simulink model "plant_1"  (R2017b)
settings: Solver=FixedStepAuto  StartTime=0.0  StopTime=10.0  FixedStep=10e-4
settings Model: Creator=Mehmet  LastModifiedBy=Mehmet

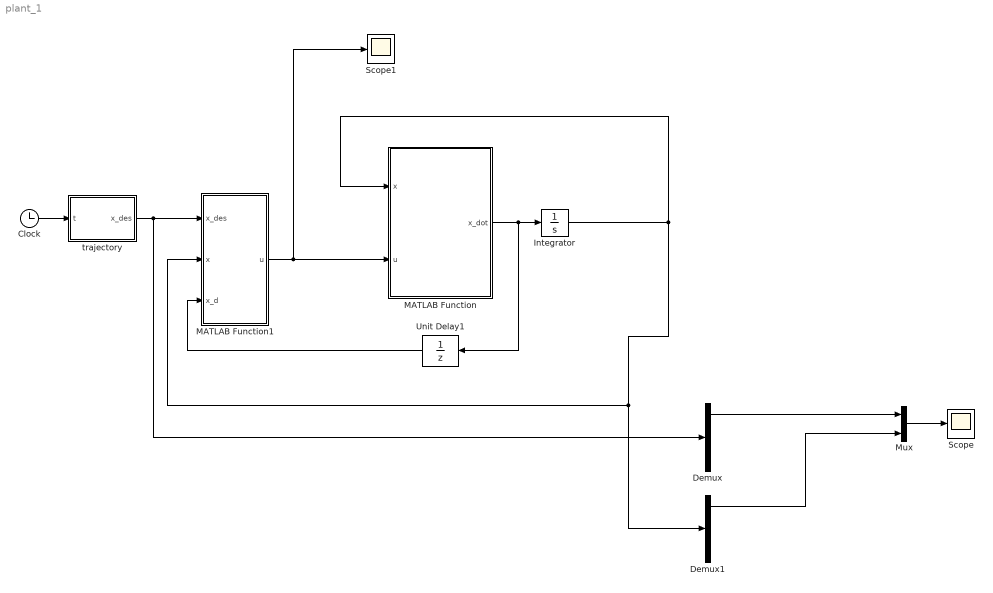
== system plant_1 ==
  Clock : Clock
  Demux : Demux  Outputs=3
  Demux1 : Demux  Outputs=3
  Integrator : Integrator  InitialCondition=[0;0;0]
  MATLAB Function : MATLAB Function  TreatAsAtomicUnit=on
  MATLAB Function1 : MATLAB Function  TreatAsAtomicUnit=on
  Mux : Mux  Inputs=2
  Scope : Scope
  Scope1 : Scope
  Unit Delay1 : UnitDelay  SampleTime=-1
  trajectory : MATLAB Function  TreatAsAtomicUnit=on
  wires:
  MATLAB Function1/1(u) -> Scope1/1, MATLAB Function/2(u)
  Clock/1 -> trajectory/1(t)
  trajectory/1(x_des) -> Demux/1, MATLAB Function1/1(x_des)
  Demux/1 -> Mux/1
  Demux1/1 -> Mux/2
  Mux/1 -> Scope/1
  MATLAB Function/1(x_dot) -> Unit Delay1/1, Integrator/1
  Integrator/1 -> Demux1/1, MATLAB Function1/2(x), MATLAB Function/1(x)
  Unit Delay1/1 -> MATLAB Function1/3(x_d)

== matlab function plant_1/MATLAB Function1 ==
  data: x_des input; u output; x input; x_d input
function u = fcn(x_des,x,x_d)

f_x = sin(x(1)) + x(2)*x(3) + x(1)*x(2)^2;
g_x = 1 + x(1)^2;

Kp = 100;
Kd = 14.14;

% v = y_dd + Kd*e_d + Kp*e;

e = x_des(1) - x(1);
e_d = x_des(2) - x_d(1);

v = x_des(3) + Kd*e_d + Kp*e;

u = 1/g_x*(-f_x + v);

end

== matlab function plant_1/MATLAB Function ==
  data: x input; u input; x_dot output
function x_dot = fcn(x,u)

q = zeros(3,1);

q(1) = x(1)*x(2) + x(3);
q(2) = -2*x(2) + x(1)*u(1);
q(3) = sin(x(1)) + 2*x(1)*x(2) + u(1);

x_dot = q;

end

== matlab function plant_1/trajectory ==
  data: t input; x_des output
function x_des = fcn(t)

A = 1;
f = 1;
w = 2*pi*f;

y = A*sin(w*t);
y_d = A*w*cos(w*t);
y_dd = -A*w*w*sin(w*t);

x_des = [y y_d y_dd]';

end
